simulink model "datatypedemo"  (R2019b)
settings: Solver=FixedStepDiscrete  StartTime=0.0  StopTime=10  FixedStep=0.01  RelTol=1e-3
PostLoadFcn:
  | hBd = get_param(bdroot, 'Handle');
  | hBlks = find_system(hBd, 'Regexp', 'on', ...
  |                               'OutDataTypeStr', 'fixdt*');
  | hLines = find_system(hBd, 'Findall', 'on', 'Regexp', 'on', ...
  |                                'Type', 'line', 'Name', 'Fixed Point*');
  | 
  | % Check that model contains expected blocks & signals
  | assert(isequal(size(hBlks), [2 1]));
  | assert(isequal(size(hLines), [2 1]));
  | 
  | if (license('test', 'fixed_point_toolbox') == 0)
  |   disp('Replacing fixed-point signals with single-precision signals')
  |   for idx = 1:length(hBlks)
  |     set_param(hBlks(idx), 'OutDataTypeStr', 'single');
  |     set_param(hLines(idx), 'Name', 'Single (fixed-point not available)');
  |   end
  | end
undefined symbols (not defined in the file): SlDemoSign
libraries: simulink x3
Description:
  | Data Typing in Simulink
  | 
  | This example shows how to use data types in Simulink.  The model used in this
  | example converts a double-precision sine wave having an amplitude of 150 to various
  | data types and displays the converted signals on two scopes.
  | 
  | The first scope shows the original sine wave and the result of converting this signal to
  | signed and unsigned 8-bit integer data types with saturation enabled.  The bottom axes
  | show the boolean results of comparing the signed and unsigned integer values.
  | 
  | The second scope shows the original sine wave and the result of converting this signal to
  | two fixed-point data types: one high-resolution, the other lower resolution.  The bottom
  | axes show the result of mapping the sine wave to an enumerated data type
  | that indicates whether the signal is positive, negative or zero.
  | 
  | Similar data type support exists for parameters and states.  Simulink also supports other
  | integer and floating-point data types, such as, single, int16, and uint32, and fixed-point
  | types with slope/bias and wordlengths from 1 to 128 bits.  You can also define types for
  | bus signals and aliases for existing types.
  | 
  | NOTE:
  | If you do not have a license for Fixed-Point Designer(TM) then the fixed-point signals will be
  | replaced by single-precision signals.
settings Model: ExtModeTrigMode=oneshot  ExtModeArmWhenConnect=off  ExtModeAutoUpdateStatusClock=off  Creator=The MathWorks, Inc.  LastModifiedBy=bhisma
settings DataIOCC: SaveFormat=Array  SaveOutput=off  SignalLogging=off  SaveTime=off
settings OptimizationCC: BlockReduction=off  BooleanDataType=off  ExpressionDepthLimit=2147483647  InitFltsAndDblsToZero=on  LifeSpan=inf  BufferReusableBoundary=off
settings DebuggingCC: SaveWithParameterizedLinksMsg=none  SignalResolutionControl=TryResolveAllWithWarning  MultiTaskDSMMsg=warning  MultiTaskCondExecSysMsg=none  IntegerOverflowMsg=none  FcnCallInpInsideContextMsg=warning  BusObjectLabelMismatch=none  AllowSymbolicDim=off  StateNameClashWarn=warning  SFUnexpectedBacktrackingDiag=warning  SFNoUnconditionalDefaultTransitionDiag=warning  SFExecutionAtInitializationDiag=none  IntegerSaturationMsg=none  ArithmeticOperatorsInVariantConditions=warning
settings HardwareCC: ProdBitPerPointer=32  ProdBitPerSizeT=32  ProdBitPerPtrDiffT=32  ProdLargestAtomicFloat=None  ProdIntDivRoundTo=Undefined  ProdEndianess=Unspecified  ProdWordSize=32  ProdHWDeviceType=32-bit Generic  TargetUnknown=on
settings ModelReferenceCC: PropagateSignalLabelsOutOfModel=off
settings SFSimCC: SimUseLocalCustomCode=off  CustomCodeUndefinedFunction=UseInterfaceOnly
settings RTWCC: Description=Generic Real-Time Target  RTWUseLocalCustomCode=off
settings CodeAppCC: StateflowObjectComments=on
settings GRTTargetCC: TargetFcnLib=ansi_tfl_tmw.mat  TargetLangStandard=C89/C90 (ANSI)  GeneratePreprocessorConditionals=Disable all  CombineOutputUpdateFcns=off  GRTInterface=on
settings ConfigComp: CovMetricSettings=dw  CovHtmlReporting=on  CovSaveCumulativeToWorkspaceVar=on  CovSaveSingleToWorkspaceVar=on  CovExternalEMLEnable=off

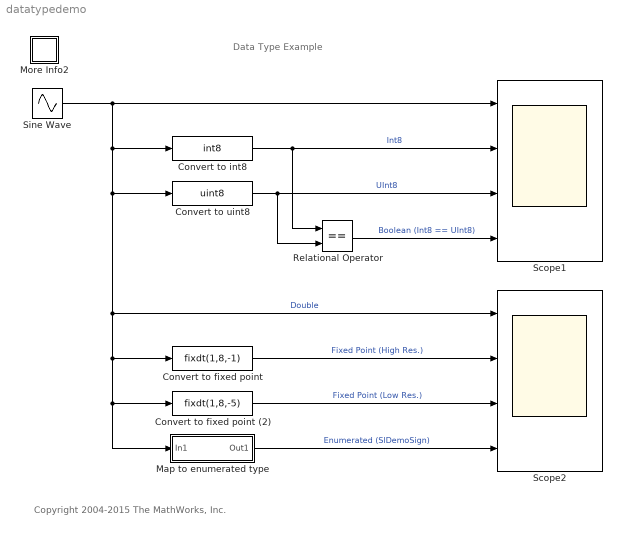
== system datatypedemo ==
  note: Data Type Example
  note: Copyright 2004-2015 The MathWorks, Inc.
  Convert to fixed point : DataTypeConversion  OutMin=-150  OutMax=150  OutDataTypeStr=fixdt(1,8,-1)  RndMeth=Zero
  Convert to fixed point (2) : DataTypeConversion  OutMin=-150  OutMax=150  OutDataTypeStr=fixdt(1,8,-5)  RndMeth=Zero
  Convert to int8 : DataTypeConversion  OutDataTypeStr=int8  SaturateOnIntegerOverflow=on  RndMeth=Zero
  Convert to uint8 : DataTypeConversion  OutDataTypeStr=uint8  SaturateOnIntegerOverflow=on  RndMeth=Zero
  Map to enumerated type : Subsystem
  More Info2 : Subsystem
      settings: OpenFcn=showdemo(bdroot(gcs))
      mask Display: disp('?')
  Relational Operator : RelationalOperator  Operator===  OutDataTypeStr=boolean  RndMeth=Nearest
  Scope1 : Scope  NumInputPorts=4
      settings: StartFcn=open_system(gcbh)
  Scope2 : Scope  NumInputPorts=4
      settings: StartFcn=open_system(gcbh)
  Sine Wave : Sin  Amplitude=150  SampleTime=0.01
  wires:
  Convert to fixed point/1 -> Scope2/2  "Fixed Point (High Res.)"
  Sine Wave/1 -> Scope1/1, Convert to int8/1, Convert to uint8/1, Convert to fixed point/1, Map to enumerated type/1(In1), Convert to fixed point (2)/1, Scope2/1  "Double"
  Convert to int8/1 -> Relational Operator/1, Scope1/2  "Int8"
  Map to enumerated type/1(Out1) -> Scope2/4  "Enumerated (SlDemoSign)"
  Convert to uint8/1 -> Relational Operator/2, Scope1/3  "UInt8"
  Relational Operator/1 -> Scope1/4  "Boolean (Int8 == UInt8)"
  Convert to fixed point (2)/1 -> Scope2/3  "Fixed Point (Low Res.)"

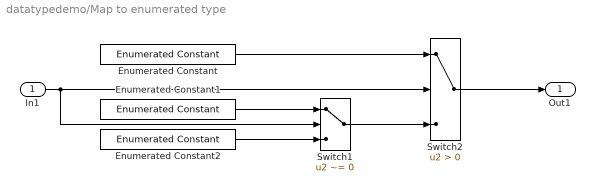
== system datatypedemo/Map to enumerated type ==
  In1 : Inport
  Enumerated Constant : simulink/Sources/Enumerated Constant  OutDataTypeStr=Enum: SlDemoSign  Value=SlDemoSign.Positive  SampleTime=Inf
      settings: SourceProductName=Simulink
  Enumerated Constant1 : simulink/Sources/Enumerated Constant  OutDataTypeStr=Enum: SlDemoSign  Value=SlDemoSign.Negative  SampleTime=Inf
      settings: SourceProductName=Simulink
  Enumerated Constant2 : simulink/Sources/Enumerated Constant  OutDataTypeStr=Enum: SlDemoSign  Value=SlDemoSign.Zero  SampleTime=Inf
      settings: SourceProductName=Simulink
  Switch1 : Switch  Criteria=u2 ~= 0
  Switch2 : Switch  Criteria=u2 > Threshold
  Out1 : Outport  VectorParamsAs1DForOutWhenUnconnected=off
  wires:
  Enumerated Constant1/1 -> Switch1/1
  Enumerated Constant2/1 -> Switch1/3
  Enumerated Constant/1 -> Switch2/1
  Switch1/1 -> Switch2/3
  In1/1 -> Switch2/2, Switch1/2
  Switch2/1 -> Out1/1

== system datatypedemo/More Info2 ==
